simulink model "Testes_Malha_LateroDircional"  (R2013b)
settings: Solver=ode45  StartTime=0.0  StopTime=10  RelTol=1e-3
values from neighbouring files (symbols this model uses):
  A = zeros(n, n)    [Lineariza.m]    (also in MatrizesDeEstado.mat = [-0.0193051557459 -0.000253889151844 -1.42063941966e-10 0 0 ; SimulacaoLinear.m = A(1:12,1:12); comparacao_paper.m = An; teste_Controlador_LateroDirecional.m = A_lat{k})
  B = zeros(n, mm)    [Lineariza.m]    (also in MatrizesDeEstado.mat = [0 0 0 0 0 0 0 0 0 0 0 0 ... (52 elements, 13x4)]; SimulacaoLinear.m = B(1:12, 2:end); comparacao_paper.m = Bn; teste_Controlador_LateroDirecional.m = B_lat{k})
  C = zeros(saidas, n)    [Lineariza.m]    (also in MatrizesDeEstado.mat = [0 0.00398133423863 0.00398133423863 0 16.2830679635 16.2830; SimulacaoLinear.m = eye(max(size(A))); comparacao_paper.m = Cn; teste_Controlador_LateroDirecional.m = [0 1 0 0)
  D = zeros(saidas, mm)    [Lineariza.m]    (also in MatrizesDeEstado.mat = [0  0  0  0; 0  -0.0485273813531  0  0; 0  -0.0485273813531 ; SimulacaoLinear.m = zeros(12,3); comparacao_paper.m = Dn; teste_Controlador_LateroDirecional.m = [0 0)
  k_i = T.Blocks.ki.Value    [comparacao_paper.m]
  k_p = T.Blocks.kp.Value    [comparacao_paper.m]
undefined symbols (not defined in the file or in its folder): k_1, k_2
settings Model: Creator=Eduardo  LastModifiedBy=Eduardo

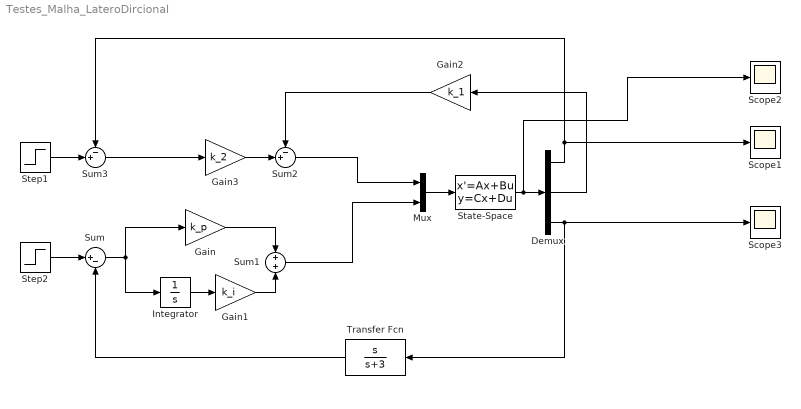
== system Testes_Malha_LateroDircional ==
  Demux : Demux  Outputs=3
  Gain : Gain  Gain=k_p
  Gain1 : Gain  Gain=k_i
  Gain2 : Gain  Gain=k_1
  Gain3 : Gain  Gain=k_2
  Integrator : Integrator
  Mux : Mux  Inputs=2
  Scope1 : Scope
  Scope2 : Scope
      settings: SaveName=ScopeData2
  Scope3 : Scope
  State-Space : StateSpace  A=A  B=B  C=C  D=D  X0=0
  Step1 : Step  SampleTime=0
  Step2 : Step  After=0  SampleTime=0
  Sum : Sum  Inputs=|+-
  Sum1 : Sum  Inputs=+|+
  Sum2 : Sum  Inputs=-+|
  Sum3 : Sum  Inputs=-+|
  Transfer Fcn : TransferFcn  Numerator=[1 0]  Denominator=[1 3]
  wires:
  Integrator/1 -> Gain1/1
  Gain/1 -> Sum1/1
  Gain1/1 -> Sum1/2
  Gain2/1 -> Sum2/1
  Sum3/1 -> Gain3/1
  Gain3/1 -> Sum2/2
  State-Space/1 -> Demux/1, Scope2/1
  Step1/1 -> Sum3/2
  Step2/1 -> Sum/1
  Sum/1 -> Gain/1, Integrator/1
  Demux/1 -> Scope1/1, Sum3/1
  Demux/2 -> Gain2/1
  Demux/3 -> Scope3/1, Transfer Fcn/1
  Mux/1 -> State-Space/1
  Sum2/1 -> Mux/1
  Sum1/1 -> Mux/2
  Transfer Fcn/1 -> Sum/2
